simulink model "SimulinkSysteme"  (Simulink 7.9)
settings: Solver=ode45  StartTime=0.0  StopTime=tsimu  RelTol=1e-3
values from neighbouring files (symbols this model uses):
  A =     [donnees_et_modeles_lineaires.mat]    (also in lmi_feedback_state_BASICS.m = [0 1 ; 5 -4]; stabilite_lmi.m = A_lin_a)
  B =     [donnees_et_modeles_lineaires.mat]    (also in lmi_feedback_state_BASICS.m = [0 ; 1]; stabilite_lmi.m = B_lin_a(:,1))
  C =     [donnees_et_modeles_lineaires.mat]
  isong = [20000 21000 22000 23000 24000 25000 26000 27000 28000 29000 30000 31000 ... (16 elements, 16x1)]    [donnees_et_modeles_lineaires.mat]    (also in donnees_turbine_v2007a.mat)
  isowf = [40 80 120 160 200 240 280 320 360 400 440 480 ... (15 elements, 15x1)]    [donnees_et_modeles_lineaires.mat]    (also in donnees_turbine_v2007a.mat)
  ntlnom = 22800    [donnees_et_modeles_lineaires.mat]    (also in donnees_turbine_v2007a.mat)
  tcg = [-4.72566699982 -2.1958899498 0.325212001801 2.65510463715 5.70554542542 9.11180782318 12.5180749893 15.9243402481 19.3306007385 22.7368736267 26.1431350708 29.5494003296 ... (240 elements, 15x16)]    [donnees_et_modeles_lineaires.mat]    (also in donnees_turbine_v2007a.mat)
  tctl100 = [-0.0806421041489 -0.00261628627777 0.383603572845 0.214125156403 0.554617404938 0.27828836441 0.00195932388306 -0.274368286133 -0.55069732666 -0.827028751373 -1.10335540771 -1.37968444824 ... (240 elements, 15x16)]    [donnees_et_modeles_lineaires.mat]    (also in donnees_turbine_v2007a.mat)
  tdctldntl = [-0.000853070175439 -0.000853070175439 -0.000853070175439 -0.000853070175439 -0.00046798245614 -0.00101842105263 -0.0012701754386 -0.00134210526316 -0.00138728070175 -0.00140219298246 -0.00144561403509 -0.00155526315789 ... (16 elements, 16x1)]    [donnees_et_modeles_lineaires.mat]    (also in donnees_turbine_v2007a.mat)
  tp3 = [1.74359560013 1.83476543427 1.89652109146 1.97084283829 2.02915382385 2.07755017281 2.12594628334 2.17434239388 2.22273850441 2.27113461494 2.31953167915 2.36792778969 ... (240 elements, 15x16)]    [donnees_et_modeles_lineaires.mat]    (also in donnees_turbine_v2007a.mat)
  tt4 = [158.323181152 257.927246094 378.081359863 509.409484863 632.046447754 753.55480957 875.063598633 996.572021484 1118.07995605 1239.58874512 1361.09716797 1482.60595703 ... (240 elements, 15x16)]    [donnees_et_modeles_lineaires.mat]    (also in donnees_turbine_v2007a.mat)
undefined symbols (not defined in the file or in its folder): Ig, Itot, steptime, stepvalue, vntlnom
settings Model: Creator=bmartine  LastModifiedBy=bmartine

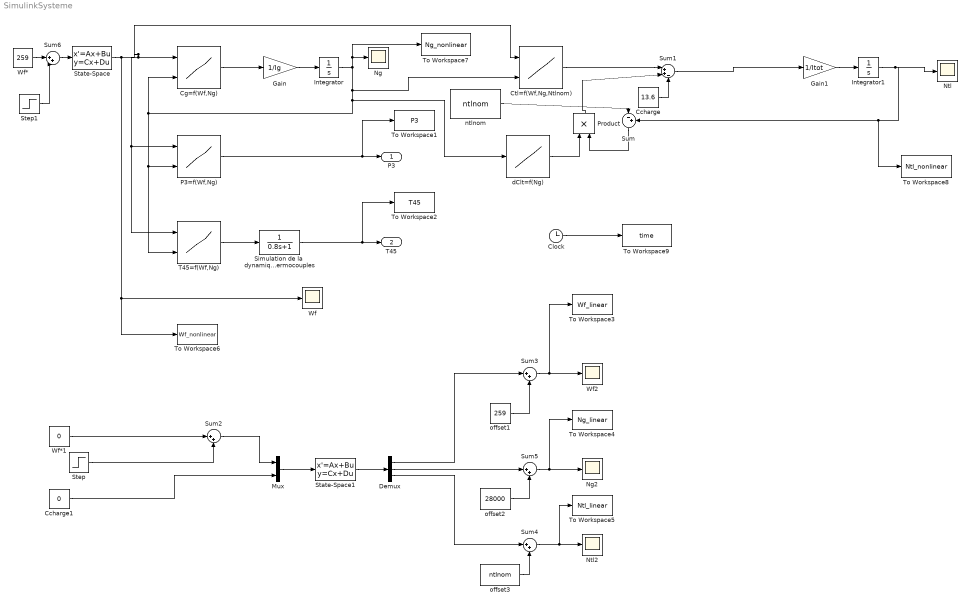
== system SimulinkSysteme ==
  Ccharge : Constant  Value=13.6
  Ccharge1 : Constant  Value=0
  Cg=f(Wf,Ng) : Lookup_n-D  BreakpointsForDimension1=isowf  BreakpointsForDimension2=isong  Table=tcg  RndMeth=Simplest  InputSameDT=on
  Clock : Clock
  Ctl=f(Wf,Ng,Ntlnom) : Lookup_n-D  BreakpointsForDimension1=isowf  BreakpointsForDimension2=isong  BreakpointsForDimension3=vntlnom  Table=tctl100  RndMeth=Simplest  InputSameDT=on
  Demux : Demux  Outputs=3
  Gain : Gain  Gain=1/Ig
  Gain1 : Gain  Gain=1/Itot
  Integrator : Integrator
  Integrator1 : Integrator  InitialCondition=ntlnom
  Mux : Mux  Inputs=2
  Ng : Scope
  Ng2 : Scope
      settings: TimeRange=10  YMin=0  YMax=8000  SaveName=ScopeData3
  Ntl : Scope
      settings: SaveName=ScopeData2
  Ntl2 : Scope
      settings: SaveName=ScopeData4
  P3=f(Wf,Ng) : Lookup_n-D  BreakpointsForDimension1=isowf  BreakpointsForDimension2=isong  Table=tp3  RndMeth=Simplest  InputSameDT=on
  Product : Product  RndMeth=Zero
  Simulation de la  dynamique des thermocouples : TransferFcn  Denominator=[0.8 1]
  State-Space : StateSpace  A=-18.52  B=4  C=4.63  D=0  X0=259
  State-Space1 : StateSpace  A=A  B=B  C=C  D=[0 0 ; 0 0 ; 0 0]
  Step : Step  Time=steptime  After=stepvalue  SampleTime=0
  Step1 : Step  Time=steptime  After=stepvalue  SampleTime=0
  Sum : Sum  Inputs=|-+
  Sum1 : Sum  Inputs=|++-
  Sum{2..6} (5 alike) : Sum  Inputs=|++
  T45=f(Wf,Ng) : Lookup_n-D  BreakpointsForDimension1=isowf  BreakpointsForDimension2=isong  Table=tt4  RndMeth=Simplest  InputSameDT=on
  To Workspace1 : ToWorkspace  VariableName=P3  SampleTime=-1
  To Workspace2 : ToWorkspace  VariableName=T45  SampleTime=-1
  To Workspace3 : ToWorkspace  VariableName=Wf_linear  SampleTime=-1
  To Workspace4 : ToWorkspace  VariableName=Ng_linear  SampleTime=-1
  To Workspace5 : ToWorkspace  VariableName=Ntl_linear  SampleTime=-1
  To Workspace6 : ToWorkspace  VariableName=Wf_nonlinear  SampleTime=-1
  To Workspace7 : ToWorkspace  VariableName=Ng_nonlinear  SampleTime=-1
  To Workspace8 : ToWorkspace  VariableName=Ntl_nonlinear  SampleTime=-1
  To Workspace9 : ToWorkspace  VariableName=time  SampleTime=-1
  Wf : Scope
  Wf* : Constant  Value=259
  Wf*1 : Constant  Value=0
  Wf2 : Scope
      settings: TimeRange=900  YMin=259.9989  YMax=259.9999  SaveName=ScopeData5
  dClt=f(Ng) : Lookup_n-D  NumberOfTableDimensions=1  BreakpointsForDimension1=isong  BreakpointsForDimension2=isong  BreakpointsForDimension3=ntlnom  Table=tdctldntl  RndMeth=Simplest  InputSameDT=on
  ntlnom : Constant  Value=ntlnom
  offset1 : Constant  Value=259
  offset2 : Constant  Value=28000
  offset3 : Constant  Value=ntlnom
  P3 : Outport
  T45 : Outport  Port=2
  wires:
  Cg=f(Wf,Ng)/1 -> Gain/1
  Gain/1 -> Integrator/1
  Integrator/1 -> Ctl=f(Wf,Ng,Ntlnom)/2, Cg=f(Wf,Ng)/2, P3=f(Wf,Ng)/2, T45=f(Wf,Ng)/2, dClt=f(Ng)/1, Ng/1, To Workspace7/1
  P3=f(Wf,Ng)/1 -> P3/1, To Workspace1/1
  T45=f(Wf,Ng)/1 -> Simulation de la  dynamique des thermocouples/1
  Simulation de la  dynamique des thermocouples/1 -> T45/1, To Workspace2/1
  ntlnom/1 -> Sum/1
  Gain1/1 -> Integrator1/1
  Integrator1/1 -> Ntl/1, Sum/2, To Workspace8/1
  Sum/1 -> Product/2
  dClt=f(Ng)/1 -> Product/1
  Product/1 -> Sum1/2
  Ctl=f(Wf,Ng,Ntlnom)/1 -> Sum1/1
  Ccharge/1 -> Sum1/3
  Sum1/1 -> Gain1/1
  State-Space/1 -> Cg=f(Wf,Ng)/1, P3=f(Wf,Ng)/1, T45=f(Wf,Ng)/1, Ctl=f(Wf,Ng,Ntlnom)/1, Wf/1, To Workspace6/1
  Mux/1 -> State-Space1/1
  Ccharge1/1 -> Mux/2
  State-Space1/1 -> Demux/1
  Wf*1/1 -> Sum2/1
  Step/1 -> Sum2/2
  Sum2/1 -> Mux/1
  Sum5/1 -> Ng2/1, To Workspace4/1
  Sum3/1 -> Wf2/1, To Workspace3/1
  Sum4/1 -> Ntl2/1, To Workspace5/1
  offset3/1 -> Sum4/2
  offset2/1 -> Sum5/2
  offset1/1 -> Sum3/2
  Demux/1 -> Sum3/1
  Demux/2 -> Sum5/1
  Demux/3 -> Sum4/1
  Clock/1 -> To Workspace9/1
  Sum6/1 -> State-Space/1
  Wf*/1 -> Sum6/1
  Step1/1 -> Sum6/2
